simulink model "P_RLC"  (R2024b)
settings: Solver=VariableStepAuto  StartTime=0.0  StopTime=.06  MaxStep=1e-4  RelTol=1e-3
values from neighbouring files (symbols this model uses):
  C = 1e-3    (= 0.001)    [defvars.m]
  L = 0.1    [defvars.m]
  R = 10    [defvars.m]
  RL = 1    [defvars.m]
settings Model: Creator=marc.nicoller  LastModifiedBy=marc.nicoller

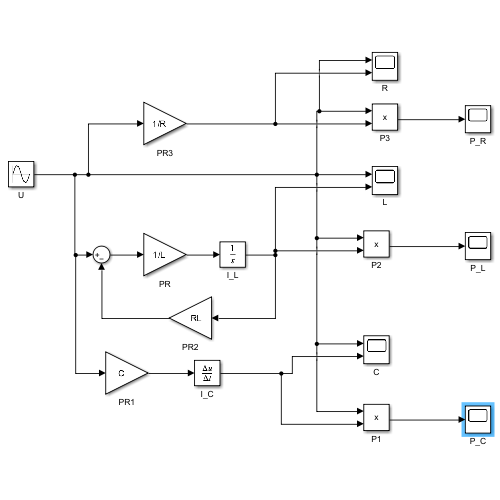
[thumbnail: Simulink's stored preview of the top-level diagram]
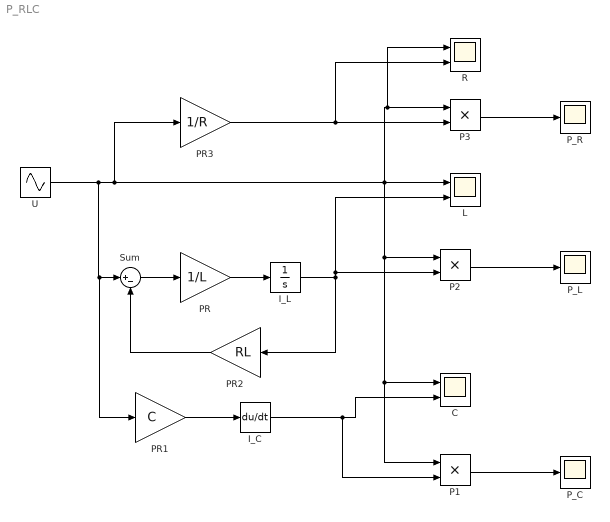
== system P_RLC ==
  C : Scope  NumInputPorts=2
  I_C : Derivative
  I_L : Integrator  InitialCondition=-230*sqrt(2)/(2*pi*L*50)
  L : Scope  NumInputPorts=2
  P1 : Product
  P2 : Product
  P3 : Product
  PR : Gain  Gain=1/L
  PR1 : Gain  Gain=C
  PR2 : Gain  Gain=RL
  PR3 : Gain  Gain=1/R
  P_C : Scope
  P_L : Scope
  P_R : Scope
  R : Scope  NumInputPorts=2
  Sum : Sum  Inputs=|+-
  U : Sin  Amplitude=230*sqrt(2)  Frequency=2*pi*50  SampleTime=0
  wires:
  PR/1 -> I_L/1
  I_L/1 -> PR2/1, P2/2, L/2
  P2/1 -> P_L/1
  PR1/1 -> I_C/1
  P1/1 -> P_C/1
  I_C/1 -> P1/2, C/2
  PR2/1 -> Sum/2
  Sum/1 -> PR/1
  PR3/1 -> R/2, P3/2
  U/1 -> Sum/1, PR1/1, PR3/1, R/1, P3/1, P2/1, P1/1, C/1, L/1
  P3/1 -> P_R/1
